simulink model "niof_model"  (R2021a)
settings: Solver=ode23tb  StartTime=0.0  StopTime=2  RelTol=1e-3
values from neighbouring files (symbols this model uses):
  h0 = ds.DateTime(1).Hour + ds.DateTime(1).Minute/60    [compiler_niof_model.m]
  S_area_hole = 0.01    [set_params_blocks.m]
undefined symbols (not defined in the file or in its folder): crop_GH1_NFT_slot1___C, crop_GH1_NFT_slot1___N, crop_GH1_NFT_slot1___R, crop_GH1_NFT_slot2___C, crop_GH1_NFT_slot2___N, crop_GH1_NFT_slot2___R, crop_GH1_NFT_slot3___C, crop_GH1_NFT_slot3___N, crop_GH1_NFT_slot3___R, crop_GH1_NFT_slot4___C, crop_GH1_NFT_slot4___N, crop_GH1_NFT_slot4___R, crop_GH1_RF_slot1___C, crop_GH1_RF_slot1___N, crop_GH1_RF_slot1___R, crop_GH1_RF_slot2___C, crop_GH1_RF_slot2___N, crop_GH1_RF_slot2___R, crop_GH1_RF_slot3___C, crop_GH1_RF_slot3___N, crop_GH1_RF_slot3___R, crop_GH1_RF_slot4___C, crop_GH1_RF_slot4___N, crop_GH1_RF_slot4___R, crop_GH2_RF_slot1___C, crop_GH2_RF_slot1___N, crop_GH2_RF_slot1___R, crop_GH2_RF_slot2___C, crop_GH2_RF_slot2___N, crop_GH2_RF_slot2___R, crop_GH2_RF_slot3___C, crop_GH2_RF_slot3___N, crop_GH2_RF_slot3___R, crop_GH2_RF_slot4___C, crop_GH2_RF_slot4___N, crop_GH2_RF_slot4___R, crop_GH2_TRAD_slot1___C, crop_GH2_TRAD_slot1___N, crop_GH2_TRAD_slot1___R, crop_GH2_TRAD_slot2___C, crop_GH2_TRAD_slot2___N, crop_GH2_TRAD_slot2___R, crop_GH2_TRAD_slot3___C, crop_GH2_TRAD_slot3___N, crop_GH2_TRAD_slot3___R, crop_GH2_TRAD_slot4___C, crop_GH2_TRAD_slot4___N, crop_GH2_TRAD_slot4___R, fish, GH3_Tank1_tend, GH3_Tank2_tend, GH3_Tank3_tend, GH3_Tank4_tend, tp_biofilter___T, tp_fish_C___T, tp_fish_M___T, tp_fish_S___T, tp_fish_T___T, tp_GH1_bio___T, tp_GH1_NFT___T ... (+3)
libraries: HORTISIM x152
(part 2 of 4)

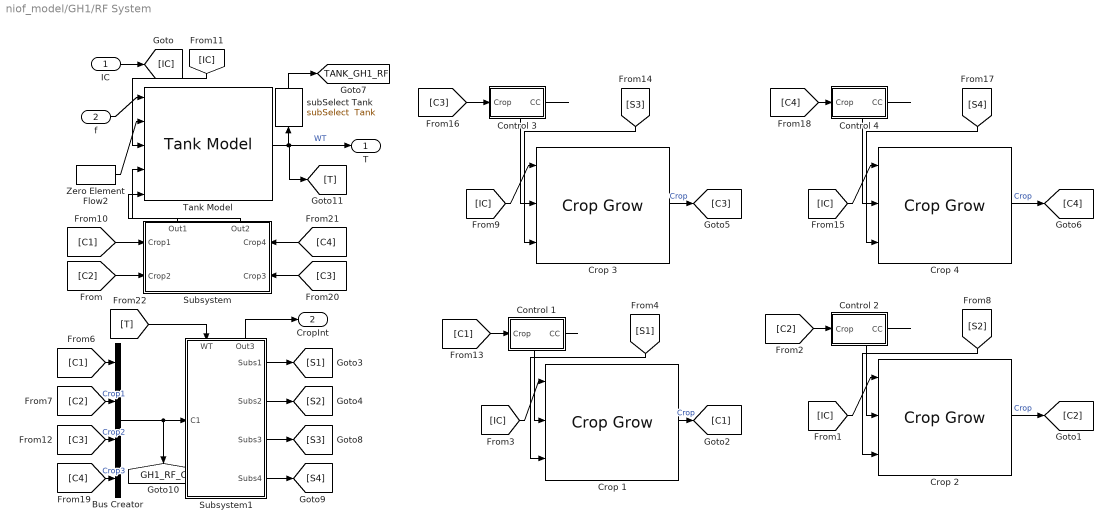
== system niof_model/GH1/RF System ==
  IC : Inport
  f : Inport  Port=2
  Bus Creator : BusCreator  Inputs=4
  Control 1 : Subsystem
  Control 2 : Subsystem
  Control 3 : Subsystem
  Control 4 : Subsystem
  Crop 1 : HORTISIM/Horticulture/Models/Crop Grow  Chi_nutrients=crop_GH1_RF_slot1___Chi_nutrients  A_v=crop_GH1_RF_slot1___A_v  plants_density=crop_GH1_RF_slot1___plants_density  fraction_DM=crop_GH1_RF_slot1___fraction_DM  min_water_capacity=crop_GH1_RF_slot1___min_water_capacity  C_buf_max=crop_GH1_RF_slot1___C_buf_max  T_v_start_fruit=crop_GH1_RF_slot1___T_v_start_fruit  int_air_speed=crop_GH1_RF_slot1___int_air_speed  b_N_uptake=crop_GH1_RF_slot1___b_N_uptake  Tv=crop_GH1_RF_slot1___Tv  C=crop_GH1_RF_slot1___C  R=crop_GH1_RF_slot1___R  Tsum=crop_GH1_RF_slot1___Tsum  C_wv=crop_GH1_RF_slot1___C_wv  N=crop_GH1_RF_slot1___N  rg_fruit=crop_GH1_RF_slot1___rg_fruit  c_fruit_m=crop_GH1_RF_slot1___c_fruit_m  c_fruit_g=crop_GH1_RF_slot1___c_fruit_g  rg_leaf=crop_GH1_RF_slot1___rg_leaf  c_leaf_m=crop_GH1_RF_slot1___c_leaf_m  c_leaf_g=crop_GH1_RF_slot1___c_leaf_g  rg_stem=crop_GH1_RF_slot1___rg_stem  c_stem_m=crop_GH1_RF_slot1___c_stem_m  c_stem_g=crop_GH1_RF_slot1___c_stem_g  VelocityAbsortion=crop_GH1_RF_slot1___VelocityAbsortion  T_max_v=crop_GH1_RF_slot1___T_max_v  s_max_T=crop_GH1_RF_slot1___s_max_T  s_min_T=crop_GH1_RF_slot1___s_min_T  s_buforg_buf=crop_GH1_RF_slot1___s_buforg_buf  T_sum_end=crop_GH1_RF_slot1___T_sum_end  T_max_v24=crop_GH1_RF_slot1___T_max_v24  T_min_v24=crop_GH1_RF_slot1___T_min_v24  s_min_T24=crop_GH1_RF_slot1___s_min_T24  s_max_T24=crop_GH1_RF_slot1___s_max_T24  T_min_v=crop_GH1_RF_slot1___T_min_v
      settings: SourceProductName=Horti Simulator
  Crop 2 : HORTISIM/Horticulture/Models/Crop Grow  Chi_nutrients=crop_GH1_RF_slot2___Chi_nutrients  A_v=crop_GH1_RF_slot2___A_v  plants_density=crop_GH1_RF_slot2___plants_density  fraction_DM=crop_GH1_RF_slot2___fraction_DM  min_water_capacity=crop_GH1_RF_slot2___min_water_capacity  C_buf_max=crop_GH1_RF_slot2___C_buf_max  T_v_start_fruit=crop_GH1_RF_slot2___T_v_start_fruit  int_air_speed=crop_GH1_RF_slot2___int_air_speed  b_N_uptake=crop_GH1_RF_slot2___b_N_uptake  Tv=crop_GH1_RF_slot2___Tv  C=crop_GH1_RF_slot2___C  R=crop_GH1_RF_slot2___R  Tsum=crop_GH1_RF_slot2___Tsum  C_wv=crop_GH1_RF_slot2___C_wv  N=crop_GH1_RF_slot2___N  rg_fruit=crop_GH1_RF_slot2___rg_fruit  c_fruit_m=crop_GH1_RF_slot2___c_fruit_m  c_fruit_g=crop_GH1_RF_slot2___c_fruit_g  rg_leaf=crop_GH1_RF_slot2___rg_leaf  c_leaf_m=crop_GH1_RF_slot2___c_leaf_m  c_leaf_g=crop_GH1_RF_slot2___c_leaf_g  rg_stem=crop_GH1_RF_slot2___rg_stem  c_stem_m=crop_GH1_RF_slot2___c_stem_m  c_stem_g=crop_GH1_RF_slot2___c_stem_g  VelocityAbsortion=crop_GH1_RF_slot2___VelocityAbsortion  T_max_v=crop_GH1_RF_slot2___T_max_v  s_max_T=crop_GH1_RF_slot2___s_max_T  s_min_T=crop_GH1_RF_slot2___s_min_T  s_buforg_buf=crop_GH1_RF_slot2___s_buforg_buf  T_sum_end=crop_GH1_RF_slot2___T_sum_end  T_max_v24=crop_GH1_RF_slot2___T_max_v24  T_min_v24=crop_GH1_RF_slot2___T_min_v24  s_min_T24=crop_GH1_RF_slot2___s_min_T24  s_max_T24=crop_GH1_RF_slot2___s_max_T24  T_min_v=crop_GH1_RF_slot2___T_min_v
      settings: SourceProductName=Horti Simulator
  Crop 3 : HORTISIM/Horticulture/Models/Crop Grow  Chi_nutrients=crop_GH1_RF_slot3___Chi_nutrients  A_v=crop_GH1_RF_slot3___A_v  plants_density=crop_GH1_RF_slot3___plants_density  fraction_DM=crop_GH1_RF_slot3___fraction_DM  min_water_capacity=crop_GH1_RF_slot3___min_water_capacity  C_buf_max=crop_GH1_RF_slot3___C_buf_max  T_v_start_fruit=crop_GH1_RF_slot3___T_v_start_fruit  int_air_speed=crop_GH1_RF_slot3___int_air_speed  b_N_uptake=crop_GH1_RF_slot3___b_N_uptake  Tv=crop_GH1_RF_slot3___Tv  C=crop_GH1_RF_slot3___C  R=crop_GH1_RF_slot3___R  Tsum=crop_GH1_RF_slot3___Tsum  C_wv=crop_GH1_RF_slot3___C_wv  N=crop_GH1_RF_slot3___N  rg_fruit=crop_GH1_RF_slot3___rg_fruit  c_fruit_m=crop_GH1_RF_slot3___c_fruit_m  c_fruit_g=crop_GH1_RF_slot3___c_fruit_g  rg_leaf=crop_GH1_RF_slot3___rg_leaf  c_leaf_m=crop_GH1_RF_slot3___c_leaf_m  c_leaf_g=crop_GH1_RF_slot3___c_leaf_g  rg_stem=crop_GH1_RF_slot3___rg_stem  c_stem_m=crop_GH1_RF_slot3___c_stem_m  c_stem_g=crop_GH1_RF_slot3___c_stem_g  VelocityAbsortion=crop_GH1_RF_slot3___VelocityAbsortion  T_max_v=crop_GH1_RF_slot3___T_max_v  s_max_T=crop_GH1_RF_slot3___s_max_T  s_min_T=crop_GH1_RF_slot3___s_min_T  s_buforg_buf=crop_GH1_RF_slot3___s_buforg_buf  T_sum_end=crop_GH1_RF_slot3___T_sum_end  T_max_v24=crop_GH1_RF_slot3___T_max_v24  T_min_v24=crop_GH1_RF_slot3___T_min_v24  s_min_T24=crop_GH1_RF_slot3___s_min_T24  s_max_T24=crop_GH1_RF_slot3___s_max_T24  T_min_v=crop_GH1_RF_slot3___T_min_v
      settings: SourceProductName=Horti Simulator
  Crop 4 : HORTISIM/Horticulture/Models/Crop Grow  Chi_nutrients=crop_GH1_RF_slot4___Chi_nutrients  A_v=crop_GH1_RF_slot4___A_v  plants_density=crop_GH1_RF_slot4___plants_density  fraction_DM=crop_GH1_RF_slot4___fraction_DM  min_water_capacity=crop_GH1_RF_slot4___min_water_capacity  C_buf_max=crop_GH1_RF_slot4___C_buf_max  T_v_start_fruit=crop_GH1_RF_slot4___T_v_start_fruit  int_air_speed=crop_GH1_RF_slot4___int_air_speed  b_N_uptake=crop_GH1_RF_slot4___b_N_uptake  Tv=crop_GH1_RF_slot4___Tv  C=crop_GH1_RF_slot4___C  R=crop_GH1_RF_slot4___R  Tsum=crop_GH1_RF_slot4___Tsum  C_wv=crop_GH1_RF_slot4___C_wv  N=crop_GH1_RF_slot4___N  rg_fruit=crop_GH1_RF_slot4___rg_fruit  c_fruit_m=crop_GH1_RF_slot4___c_fruit_m  c_fruit_g=crop_GH1_RF_slot4___c_fruit_g  rg_leaf=crop_GH1_RF_slot4___rg_leaf  c_leaf_m=crop_GH1_RF_slot4___c_leaf_m  c_leaf_g=crop_GH1_RF_slot4___c_leaf_g  rg_stem=crop_GH1_RF_slot4___rg_stem  c_stem_m=crop_GH1_RF_slot4___c_stem_m  c_stem_g=crop_GH1_RF_slot4___c_stem_g  VelocityAbsortion=crop_GH1_RF_slot4___VelocityAbsortion  T_max_v=crop_GH1_RF_slot4___T_max_v  s_max_T=crop_GH1_RF_slot4___s_max_T  s_min_T=crop_GH1_RF_slot4___s_min_T  s_buforg_buf=crop_GH1_RF_slot4___s_buforg_buf  T_sum_end=crop_GH1_RF_slot4___T_sum_end  T_max_v24=crop_GH1_RF_slot4___T_max_v24  T_min_v24=crop_GH1_RF_slot4___T_min_v24  s_min_T24=crop_GH1_RF_slot4___s_min_T24  s_max_T24=crop_GH1_RF_slot4___s_max_T24  T_min_v=crop_GH1_RF_slot4___T_min_v
      settings: SourceProductName=Horti Simulator
  Subsystem : Subsystem
      settings: PortSchema="{\"entries\":[{\"content\":{\"sides\":[{\"content\":{\"connectorIds\":[]},\"type\":\"ConnectorPlacement.EquallySpacedRectSide\",\"uuid\":\"331b7e07-99e0-48a1-afa9-efd959d86c3c\"},{\"content\":{\"connectorIds\":[\"Out1\",\"Out2\"],\"side\":\"RIGHT\"},\"type\":\"ConnectorPlacement.EquallySpacedRectSide\",\"uuid\":\"88f560c2-c33d-415c-abbb-9cce13a50e34\"},{\"content\":{\"connectorIds\":[\"In1\",\"In2\"],\"side\":\"TOP\"},\"type\":\"ConnectorPlacement.EquallySpacedRectSide\",\"uuid\":\"5809bd20-6d1a-4a08-a3be-af6196f2651a\"},{\"content\":{\"connectorIds\":[\"In3\",\"In4\"],\"side\":\"BOTTOM\"},\"type\":\"ConnectorPlacement.EquallySpacedRectSide\",\"uuid\":\"0451beb0-e3d9-4028-a291-a4662efcb901\"}]},\"type\":\"ConnectorPlacement.EquallySpacedConnector\",\"uuid\":\"8352e301-80a0-449c-83b8-038a5d79df4c\"}],\"packageUris\":[\"http://schema.mathworks.com/mf0/Connector/R2020b\"],\"version\":\"1.0\"}"
  Subsystem1 : Subsystem
      settings: PortSchema="{\"entries\":[{\"content\":{\"sides\":[{\"content\":{\"connectorIds\":[\"In1\"]},\"type\":\"ConnectorPlacement.EquallySpacedRectSide\",\"uuid\":\"4fbee580-d560-4e1c-bbb5-c1692f8814f1\"},{\"content\":{\"connectorIds\":[\"Out1\",\"Out2\",\"Out3\",\"Out4\"],\"side\":\"RIGHT\"},\"type\":\"ConnectorPlacement.EquallySpacedRectSide\",\"uuid\":\"81a4a23d-0981-460c-8110-0a6c3dae9561\"},{\"content\":{\"connectorIds\":[\"In2\",\"Out5\"],\"side\":\"TOP\"},\"type\":\"ConnectorPlacement.EquallySpacedRectSide\",\"uuid\":\"d86bf355-ad16-490c-942f-99534b60638b\"},{\"content\":{\"connectorIds\":[],\"side\":\"BOTTOM\"},\"type\":\"ConnectorPlacement.EquallySpacedRectSide\",\"uuid\":\"eaa009ab-e9b5-48b4-8c60-43d182c3bfd7\"}]},\"type\":\"ConnectorPlacement.EquallySpacedConnector\",\"uuid\":\"d99c9aa8-04cd-4090-9f71-30da2befe22b\"}],\"packageUris\":[\"http://schema.mathworks.com/mf0/Connector/R2020b\"],\"version\":\"1.0\"}"
  Tank Model : HORTISIM/Aquaculture/Models/Tank Model  S=tp_GH1_RF___S  h_max=tp_GH1_RF___h_max  wall_gain=tp_GH1_RF___wall_gain  ThermalConductivityWall=tp_GH1_RF___ThermalConductivityWall  Tsubwall=tp_GH1_RF___Tsubwall  h=tp_GH1_RF___h  X=tp_GH1_RF___X  T=tp_GH1_RF___T  Twall=tp_GH1_RF___Twall  d_t=tp_GH1_RF___d_t
      settings: SourceProductName=Horti Simulator
  Zero Element Flow2 : HORTISIM/Other  Functions/Zero Element Flow  SystemSampleTime=-1  VariantActivationTime=update diagram  Latency=0  AutoFrameSizeCalculation=off
      settings: SourceProductName=Horti Simulator
  subSelect Tank : HORTISIM/Other  Functions/subSelect  Tank  SystemSampleTime=-1  VariantActivationTime=update diagram  Latency=0  AutoFrameSizeCalculation=off
      settings: SourceProductName=Horti Simulator
  T : Outport
  CropInt : Outport  Port=2
  tag scope: GH1_RF_C=global, TANK_GH1_RF=global
  wires:
  f/1 -> Tank Model/1
  [IC] -> Tank Model/3
  Tank Model/1 -> [T], T/1, subSelect Tank/1  "WT"
  [IC] -> Crop 1/1
  Control 1/1(CC) -> Crop 1/2
  Crop 1/1 -> [C1]  "Crop"
  Zero Element Flow2/1 -> Tank Model/2
  [C1] -> Control 1/1(Crop)
  IC/1 -> [IC]
  [IC] -> Crop 2/1
  Crop 2/1 -> [C2]  "Crop"
  [C2] -> Control 2/1(Crop)
  Control 2/1(CC) -> Crop 2/2
  [S1] -> Crop 1/3
  [S2] -> Crop 2/3
  [C1] -> Subsystem/2(Crop1)
  [C2] -> Subsystem/1(Crop2)
  Subsystem/1(Out1) -> Tank Model/4
  Subsystem/2(Out2) -> Tank Model/5
  [IC] -> Crop 3/1
  Crop 3/1 -> [C3]  "Crop"
  [S3] -> Crop 3/3
  [C3] -> Control 3/1(Crop)
  Control 3/1(CC) -> Crop 3/2
  [IC] -> Crop 4/1
  Crop 4/1 -> [C4]  "Crop"
  [S4] -> Crop 4/3
  [C4] -> Control 4/1(Crop)
  Control 4/1(CC) -> Crop 4/2
  [C3] -> Subsystem/3(Crop3)
  [C4] -> Subsystem/4(Crop4)
  [T] -> Subsystem1/2(WT)
  Subsystem1/1(Subs1) -> [S1]
  Subsystem1/2(Subs2) -> [S2]
  Subsystem1/5(Out3) -> CropInt/1
  Subsystem1/3(Subs3) -> [S3]
  Subsystem1/4(Subs4) -> [S4]
  [C1] -> Bus Creator/1
  [C2] -> Bus Creator/2  "Crop1"
  [C3] -> Bus Creator/3  "Crop2"
  [C4] -> Bus Creator/4  "Crop3"
  Bus Creator/1 -> [GH1_RF_C], Subsystem1/1(C1)
  subSelect Tank/1 -> [TANK_GH1_RF]

== system niof_model/GH1/Subsystem ==
  In1 : Inport
  In2 : Inport  Port=2
  In3 : Inport  Port=3
  In4 : Inport  Port=4
  Crop2ExtArray : HORTISIM/Other  Functions/Crop2ExtArray  SystemSampleTime=-1  VariantActivationTime=update diagram  Latency=0  AutoFrameSizeCalculation=off
      settings: SourceProductName=Horti Simulator
  Crop2ExtArray1 : HORTISIM/Other  Functions/Crop2ExtArray  SystemSampleTime=-1  VariantActivationTime=update diagram  Latency=0  AutoFrameSizeCalculation=off
      settings: SourceProductName=Horti Simulator
  MatrixExt2Bus : HORTISIM/Other  Functions/MatrixExt2Bus  SystemSampleTime=-1  VariantActivationTime=update diagram  Latency=0  AutoFrameSizeCalculation=off
      settings: SourceProductName=Horti Simulator
  Tank2ExtArray : HORTISIM/Other  Functions/Tank2ExtArray  SystemSampleTime=-1  VariantActivationTime=update diagram  Latency=0  AutoFrameSizeCalculation=off
      settings: SourceProductName=Horti Simulator
  Tank2ExtArray1 : HORTISIM/Other  Functions/Tank2ExtArray  SystemSampleTime=-1  VariantActivationTime=update diagram  Latency=0  AutoFrameSizeCalculation=off
      settings: SourceProductName=Horti Simulator
  Vector Concatenate : Concatenate  NumInputs=4  Mode=Multidimensional array  ConcatenateDimension=2
  CoCl : Outport
  wires:
  MatrixExt2Bus/1 -> CoCl/1
  In2/1 -> Tank2ExtArray/1
  Crop2ExtArray1/1 -> Vector Concatenate/4
  In1/1 -> Crop2ExtArray/1
  In3/1 -> Tank2ExtArray1/1
  Tank2ExtArray1/1 -> Vector Concatenate/3
  In4/1 -> Crop2ExtArray1/1
  Vector Concatenate/1 -> MatrixExt2Bus/1
  Tank2ExtArray/1 -> Vector Concatenate/2
  Crop2ExtArray/1 -> Vector Concatenate/1

== system niof_model/GH1/Subsystem1 ==
  In1 : Inport
  In2 : Inport  Port=2
  Bus Selector : BusSelector  OutputSignals=Drainge
  Bus Selector1 : BusSelector  OutputSignals=Drainge
  Subsystem3 : Subsystem
  Out1 : Outport
  wires:
  In2/1 -> Bus Selector1/1
  In1/1 -> Bus Selector/1
  Bus Selector/1 -> Subsystem3/1(In1)  "<Drainge>"
  Subsystem3/1(Out1) -> Out1/1
  Bus Selector1/1 -> Subsystem3/2(In2)  "<Drainge>"

== system niof_model/GH2/Flow2Divisor ==
  Fo2 : Inport
  In1 : Inport  Port=2
  Bus Creator : BusCreator  Inputs=3  OutDataTypeStr=Bus: FLOW  NonVirtualBus=on
  Bus Creator1 : BusCreator  Inputs=3  OutDataTypeStr=Bus: FLOW  NonVirtualBus=on
  Bus Selector : BusSelector  OutputSignals=f,T,X
  Constant : Constant
  Minus : Sum  Inputs=+-
  Product : Product
  Product1 : Product
  Out1 : Outport
  Out2 : Outport  Port=2
  wires:
  Fo2/1 -> Bus Selector/1
  Bus Selector/1 -> Product1/2, Product/2  "<f>"
  Product/1 -> [f1]
  Bus Selector/2 -> [T]  "<T>"
  Bus Selector/3 -> [X]  "<X>"
  [f1] -> Bus Creator/1  "f"
  [T] -> Bus Creator/2  "T"
  Bus Creator/1 -> Out1/1
  [X] -> Bus Creator/3  "X"
  [f2] -> Bus Creator1/1  "f"
  [T] -> Bus Creator1/2  "T"
  Bus Creator1/1 -> Out2/1
  [X] -> Bus Creator1/3  "X"
  In1/1 -> Product/1, Minus/2
  Constant/1 -> Minus/1
  Minus/1 -> Product1/1
  Product1/1 -> [f2]

== system niof_model/GH2/Mezcla Calor, Vapor de agua y CO2 desde los tanques de agua y la plantación ==
  In2 : Inport
  In3 : Inport  Port=2
  In4 : Inport  Port=3
  In1 : Inport  Port=4
  Crop2ExtArray : Subsystem  AncestorBlock="HORTISIM/Other  Functions/Crop2ExtArray"
  Crop2ExtArray1 : HORTISIM/Other  Functions/Crop2ExtArray  SystemSampleTime=-1  VariantActivationTime=update diagram  Latency=0  AutoFrameSizeCalculation=off
      settings: SourceProductName=Horti Simulator
  MatrixExt2Bus : Subsystem  AncestorBlock="HORTISIM/Other  Functions/MatrixExt2Bus"
  Tank2ExtArray : Subsystem  AncestorBlock="HORTISIM/Other  Functions/Tank2ExtArray"
  Tank2ExtArray1 : HORTISIM/Other  Functions/Tank2ExtArray  SystemSampleTime=-1  VariantActivationTime=update diagram  Latency=0  AutoFrameSizeCalculation=off
      settings: SourceProductName=Horti Simulator
  Vector Concatenate : Concatenate  NumInputs=4  Mode=Multidimensional array  ConcatenateDimension=2
  CoCl : Outport
  wires:
  In4/1 -> Crop2ExtArray1/1
  In3/1 -> Tank2ExtArray1/1
  In2/1 -> Tank2ExtArray/1(In1)
  Crop2ExtArray/1(Out1) -> Vector Concatenate/1
  Vector Concatenate/1 -> MatrixExt2Bus/1(In1)
  MatrixExt2Bus/1(CoCl) -> CoCl/1
  Tank2ExtArray/1(Out1) -> Vector Concatenate/2
  Tank2ExtArray1/1 -> Vector Concatenate/3
  Crop2ExtArray1/1 -> Vector Concatenate/4
  In1/1 -> Crop2ExtArray/1(In1)

== system niof_model/GH2/Null Element ==
  Scalar2Bus Control Climate : HORTISIM/Other  Functions/Scalar2Bus  Control Climate  SystemSampleTime=-1  VariantActivationTime=update diagram  Latency=0  AutoFrameSizeCalculation=off
      settings: SourceProductName=Horti Simulator
  Zero Element Screen : HORTISIM/Other  Functions/Zero Element Screen  SystemSampleTime=-1  VariantActivationTime=update diagram  Latency=0  AutoFrameSizeCalculation=off
      settings: SourceProductName=Horti Simulator
  Zero Element Windows : HORTISIM/Other  Functions/Zero Element Windows  SystemSampleTime=-1  VariantActivationTime=update diagram  Latency=0  AutoFrameSizeCalculation=off
      link override Constant1: Value=1
      settings: SourceProductName=Horti Simulator
  CoCl : Outport
  wires:
  Scalar2Bus Control Climate/1 -> CoCl/1
  Zero Element Windows/1 -> Scalar2Bus Control Climate/1
  ? -> Scalar2Bus Control Climate/4
  ? -> Scalar2Bus Control Climate/3
  Zero Element Screen/1 -> Scalar2Bus Control Climate/2

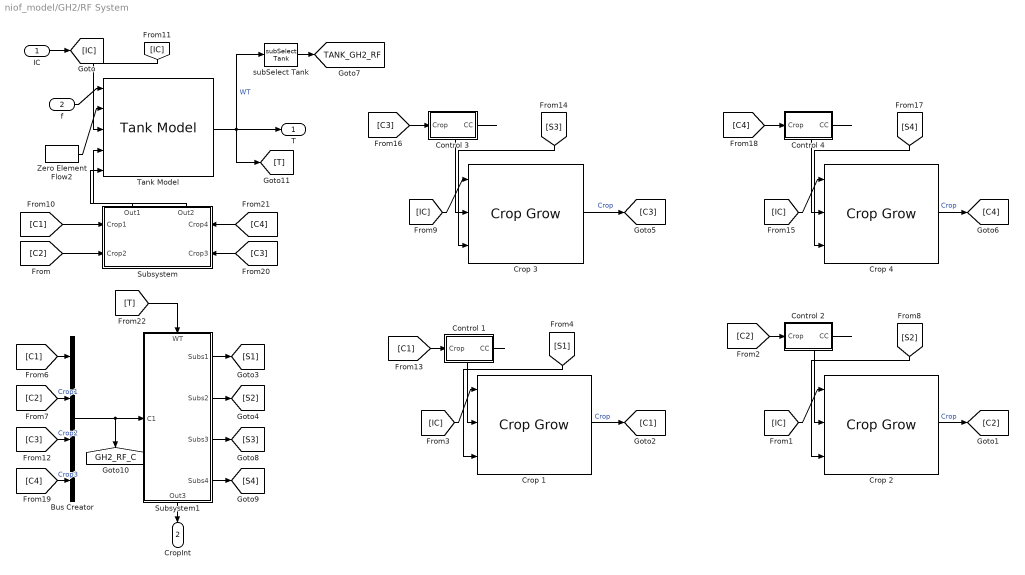
== system niof_model/GH2/RF System ==
  IC : Inport
  f : Inport  Port=2
  Bus Creator : BusCreator  Inputs=4
  Control 1 : Subsystem
  Control 2 : Subsystem
  Control 3 : Subsystem
  Control 4 : Subsystem
  Crop 1 : HORTISIM/Horticulture/Models/Crop Grow  Chi_nutrients=crop_GH2_RF_slot1___Chi_nutrients  A_v=crop_GH2_RF_slot1___A_v  plants_density=crop_GH2_RF_slot1___plants_density  fraction_DM=crop_GH2_RF_slot1___fraction_DM  min_water_capacity=crop_GH2_RF_slot1___min_water_capacity  C_buf_max=crop_GH2_RF_slot1___C_buf_max  T_v_start_fruit=crop_GH2_RF_slot1___T_v_start_fruit  int_air_speed=crop_GH2_RF_slot1___int_air_speed  b_N_uptake=crop_GH2_RF_slot1___b_N_uptake  Tv=crop_GH2_RF_slot1___Tv  C=crop_GH2_RF_slot1___C  R=crop_GH2_RF_slot1___R  Tsum=crop_GH2_RF_slot1___Tsum  C_wv=crop_GH2_RF_slot1___C_wv  N=crop_GH2_RF_slot1___N  rg_fruit=crop_GH2_RF_slot1___rg_fruit  c_fruit_m=crop_GH2_RF_slot1___c_fruit_m  c_fruit_g=crop_GH2_RF_slot1___c_fruit_g  rg_leaf=crop_GH2_RF_slot1___rg_leaf  c_leaf_m=crop_GH2_RF_slot1___c_leaf_m  c_leaf_g=crop_GH2_RF_slot1___c_leaf_g  rg_stem=crop_GH2_RF_slot1___rg_stem  c_stem_m=crop_GH2_RF_slot1___c_stem_m  c_stem_g=crop_GH2_RF_slot1___c_stem_g  VelocityAbsortion=crop_GH2_RF_slot1___VelocityAbsortion  T_max_v=crop_GH2_RF_slot1___T_max_v  s_max_T=crop_GH2_RF_slot1___s_max_T  s_min_T=crop_GH2_RF_slot1___s_min_T  s_buforg_buf=crop_GH2_RF_slot1___s_buforg_buf  T_sum_end=crop_GH2_RF_slot1___T_sum_end  T_max_v24=crop_GH2_RF_slot1___T_max_v24  T_min_v24=crop_GH2_RF_slot1___T_min_v24  s_min_T24=crop_GH2_RF_slot1___s_min_T24  s_max_T24=crop_GH2_RF_slot1___s_max_T24  T_min_v=crop_GH2_RF_slot1___T_min_v
      settings: SourceProductName=Horti Simulator
  Crop 2 : HORTISIM/Horticulture/Models/Crop Grow  Chi_nutrients=crop_GH2_RF_slot2___Chi_nutrients  A_v=crop_GH2_RF_slot2___A_v  plants_density=crop_GH2_RF_slot2___plants_density  fraction_DM=crop_GH2_RF_slot2___fraction_DM  min_water_capacity=crop_GH2_RF_slot2___min_water_capacity  C_buf_max=crop_GH2_RF_slot2___C_buf_max  T_v_start_fruit=crop_GH2_RF_slot2___T_v_start_fruit  int_air_speed=crop_GH2_RF_slot2___int_air_speed  b_N_uptake=crop_GH2_RF_slot2___b_N_uptake  Tv=crop_GH2_RF_slot2___Tv  C=crop_GH2_RF_slot2___C  R=crop_GH2_RF_slot2___R  Tsum=crop_GH2_RF_slot2___Tsum  C_wv=crop_GH2_RF_slot2___C_wv  N=crop_GH2_RF_slot2___N  rg_fruit=crop_GH2_RF_slot2___rg_fruit  c_fruit_m=crop_GH2_RF_slot2___c_fruit_m  c_fruit_g=crop_GH2_RF_slot2___c_fruit_g  rg_leaf=crop_GH2_RF_slot2___rg_leaf  c_leaf_m=crop_GH2_RF_slot2___c_leaf_m  c_leaf_g=crop_GH2_RF_slot2___c_leaf_g  rg_stem=crop_GH2_RF_slot2___rg_stem  c_stem_m=crop_GH2_RF_slot2___c_stem_m  c_stem_g=crop_GH2_RF_slot2___c_stem_g  VelocityAbsortion=crop_GH2_RF_slot2___VelocityAbsortion  T_max_v=crop_GH2_RF_slot2___T_max_v  s_max_T=crop_GH2_RF_slot2___s_max_T  s_min_T=crop_GH2_RF_slot2___s_min_T  s_buforg_buf=crop_GH2_RF_slot2___s_buforg_buf  T_sum_end=crop_GH2_RF_slot2___T_sum_end  T_max_v24=crop_GH2_RF_slot2___T_max_v24  T_min_v24=crop_GH2_RF_slot2___T_min_v24  s_min_T24=crop_GH2_RF_slot2___s_min_T24  s_max_T24=crop_GH2_RF_slot2___s_max_T24  T_min_v=crop_GH2_RF_slot2___T_min_v
      settings: SourceProductName=Horti Simulator
  Crop 3 : HORTISIM/Horticulture/Models/Crop Grow  Chi_nutrients=crop_GH2_RF_slot3___Chi_nutrients  A_v=crop_GH2_RF_slot3___A_v  plants_density=crop_GH2_RF_slot3___plants_density  fraction_DM=crop_GH2_RF_slot3___fraction_DM  min_water_capacity=crop_GH2_RF_slot3___min_water_capacity  C_buf_max=crop_GH2_RF_slot3___C_buf_max  T_v_start_fruit=crop_GH2_RF_slot3___T_v_start_fruit  int_air_speed=crop_GH2_RF_slot3___int_air_speed  b_N_uptake=crop_GH2_RF_slot3___b_N_uptake  Tv=crop_GH2_RF_slot3___Tv  C=crop_GH2_RF_slot3___C  R=crop_GH2_RF_slot3___R  Tsum=crop_GH2_RF_slot3___Tsum  C_wv=crop_GH2_RF_slot3___C_wv  N=crop_GH2_RF_slot3___N  rg_fruit=crop_GH2_RF_slot3___rg_fruit  c_fruit_m=crop_GH2_RF_slot3___c_fruit_m  c_fruit_g=crop_GH2_RF_slot3___c_fruit_g  rg_leaf=crop_GH2_RF_slot3___rg_leaf  c_leaf_m=crop_GH2_RF_slot3___c_leaf_m  c_leaf_g=crop_GH2_RF_slot3___c_leaf_g  rg_stem=crop_GH2_RF_slot3___rg_stem  c_stem_m=crop_GH2_RF_slot3___c_stem_m  c_stem_g=crop_GH2_RF_slot3___c_stem_g  VelocityAbsortion=crop_GH2_RF_slot3___VelocityAbsortion  T_max_v=crop_GH2_RF_slot3___T_max_v  s_max_T=crop_GH2_RF_slot3___s_max_T  s_min_T=crop_GH2_RF_slot3___s_min_T  s_buforg_buf=crop_GH2_RF_slot3___s_buforg_buf  T_sum_end=crop_GH2_RF_slot3___T_sum_end  T_max_v24=crop_GH2_RF_slot3___T_max_v24  T_min_v24=crop_GH2_RF_slot3___T_min_v24  s_min_T24=crop_GH2_RF_slot3___s_min_T24  s_max_T24=crop_GH2_RF_slot3___s_max_T24  T_min_v=crop_GH2_RF_slot3___T_min_v
      settings: SourceProductName=Horti Simulator
  Crop 4 : HORTISIM/Horticulture/Models/Crop Grow  Chi_nutrients=crop_GH2_RF_slot4___Chi_nutrients  A_v=crop_GH2_RF_slot4___A_v  plants_density=crop_GH2_RF_slot4___plants_density  fraction_DM=crop_GH2_RF_slot4___fraction_DM  min_water_capacity=crop_GH2_RF_slot4___min_water_capacity  C_buf_max=crop_GH2_RF_slot4___C_buf_max  T_v_start_fruit=crop_GH2_RF_slot4___T_v_start_fruit  int_air_speed=crop_GH2_RF_slot4___int_air_speed  b_N_uptake=crop_GH2_RF_slot4___b_N_uptake  Tv=crop_GH2_RF_slot4___Tv  C=crop_GH2_RF_slot4___C  R=crop_GH2_RF_slot4___R  Tsum=crop_GH2_RF_slot4___Tsum  C_wv=crop_GH2_RF_slot4___C_wv  N=crop_GH2_RF_slot4___N  rg_fruit=crop_GH2_RF_slot4___rg_fruit  c_fruit_m=crop_GH2_RF_slot4___c_fruit_m  c_fruit_g=crop_GH2_RF_slot4___c_fruit_g  rg_leaf=crop_GH2_RF_slot4___rg_leaf  c_leaf_m=crop_GH2_RF_slot4___c_leaf_m  c_leaf_g=crop_GH2_RF_slot4___c_leaf_g  rg_stem=crop_GH2_RF_slot4___rg_stem  c_stem_m=crop_GH2_RF_slot4___c_stem_m  c_stem_g=crop_GH2_RF_slot4___c_stem_g  VelocityAbsortion=crop_GH2_RF_slot4___VelocityAbsortion  T_max_v=crop_GH2_RF_slot4___T_max_v  s_max_T=crop_GH2_RF_slot4___s_max_T  s_min_T=crop_GH2_RF_slot4___s_min_T  s_buforg_buf=crop_GH2_RF_slot4___s_buforg_buf  T_sum_end=crop_GH2_RF_slot4___T_sum_end  T_max_v24=crop_GH2_RF_slot4___T_max_v24  T_min_v24=crop_GH2_RF_slot4___T_min_v24  s_min_T24=crop_GH2_RF_slot4___s_min_T24  s_max_T24=crop_GH2_RF_slot4___s_max_T24  T_min_v=crop_GH2_RF_slot4___T_min_v
      settings: SourceProductName=Horti Simulator
  Subsystem : Subsystem
      settings: PortSchema="{\"entries\":[{\"content\":{\"sides\":[{\"content\":{\"connectorIds\":[]},\"type\":\"ConnectorPlacement.EquallySpacedRectSide\",\"uuid\":\"331b7e07-99e0-48a1-afa9-efd959d86c3c\"},{\"content\":{\"connectorIds\":[\"Out1\",\"Out2\"],\"side\":\"RIGHT\"},\"type\":\"ConnectorPlacement.EquallySpacedRectSide\",\"uuid\":\"88f560c2-c33d-415c-abbb-9cce13a50e34\"},{\"content\":{\"connectorIds\":[\"In1\",\"In2\"],\"side\":\"TOP\"},\"type\":\"ConnectorPlacement.EquallySpacedRectSide\",\"uuid\":\"5809bd20-6d1a-4a08-a3be-af6196f2651a\"},{\"content\":{\"connectorIds\":[\"In3\",\"In4\"],\"side\":\"BOTTOM\"},\"type\":\"ConnectorPlacement.EquallySpacedRectSide\",\"uuid\":\"0451beb0-e3d9-4028-a291-a4662efcb901\"}]},\"type\":\"ConnectorPlacement.EquallySpacedConnector\",\"uuid\":\"8352e301-80a0-449c-83b8-038a5d79df4c\"}],\"packageUris\":[\"http://schema.mathworks.com/mf0/Connector/R2020b\"],\"version\":\"1.0\"}"
  Subsystem1 : Subsystem
      settings: PortSchema="{\"entries\":[{\"content\":{\"sides\":[{\"content\":{\"connectorIds\":[\"In1\"]},\"type\":\"ConnectorPlacement.EquallySpacedRectSide\",\"uuid\":\"4fbee580-d560-4e1c-bbb5-c1692f8814f1\"},{\"content\":{\"connectorIds\":[\"Out1\",\"Out2\",\"Out3\",\"Out4\"],\"side\":\"RIGHT\"},\"type\":\"ConnectorPlacement.EquallySpacedRectSide\",\"uuid\":\"81a4a23d-0981-460c-8110-0a6c3dae9561\"},{\"content\":{\"connectorIds\":[\"In2\"],\"side\":\"TOP\"},\"type\":\"ConnectorPlacement.EquallySpacedRectSide\",\"uuid\":\"d86bf355-ad16-490c-942f-99534b60638b\"},{\"content\":{\"connectorIds\":[\"Out5\"],\"side\":\"BOTTOM\"},\"type\":\"ConnectorPlacement.EquallySpacedRectSide\",\"uuid\":\"eaa009ab-e9b5-48b4-8c60-43d182c3bfd7\"}]},\"type\":\"ConnectorPlacement.EquallySpacedConnector\",\"uuid\":\"d99c9aa8-04cd-4090-9f71-30da2befe22b\"}],\"packageUris\":[\"http://schema.mathworks.com/mf0/Connector/R2020b\"],\"version\":\"1.0\"}"
  Tank Model : HORTISIM/Aquaculture/Models/Tank Model  S=tp_GH2_RF___S  h_max=tp_GH2_RF___h_max  wall_gain=tp_GH2_RF___wall_gain  ThermalConductivityWall=tp_GH2_RF___ThermalConductivityWall  Tsubwall=tp_GH2_RF___Tsubwall  h=tp_GH2_RF___h  X=tp_GH2_RF___X  T=tp_GH2_RF___T  Twall=tp_GH2_RF___Twall  d_t=tp_GH2_RF___d_t
      settings: SourceProductName=Horti Simulator
  Zero Element Flow2 : HORTISIM/Other  Functions/Zero Element Flow  SystemSampleTime=-1  VariantActivationTime=update diagram  Latency=0  AutoFrameSizeCalculation=off
      settings: SourceProductName=Horti Simulator
  subSelect Tank : HORTISIM/Other  Functions/subSelect  Tank  SystemSampleTime=-1  VariantActivationTime=update diagram  Latency=0  AutoFrameSizeCalculation=off
      settings: SourceProductName=Horti Simulator
  T : Outport
  CropInt : Outport  Port=2
  tag scope: GH2_RF_C=global, TANK_GH2_RF=global
  wires:
  f/1 -> Tank Model/1
  [IC] -> Tank Model/3
  Tank Model/1 -> T/1, [T], subSelect Tank/1  "WT"
  [IC] -> Crop 1/1
  Control 1/1(CC) -> Crop 1/2
  Crop 1/1 -> [C1]  "Crop"
  Zero Element Flow2/1 -> Tank Model/2
  [C1] -> Control 1/1(Crop)
  IC/1 -> [IC]
  [IC] -> Crop 2/1
  Crop 2/1 -> [C2]  "Crop"
  [C2] -> Control 2/1(Crop)
  Control 2/1(CC) -> Crop 2/2
  [S1] -> Crop 1/3
  [S2] -> Crop 2/3
  [C1] -> Subsystem/2(Crop1)
  [C2] -> Subsystem/1(Crop2)
  Subsystem/1(Out1) -> Tank Model/4
  Subsystem/2(Out2) -> Tank Model/5
  [IC] -> Crop 3/1
  Crop 3/1 -> [C3]  "Crop"
  [S3] -> Crop 3/3
  [C3] -> Control 3/1(Crop)
  Control 3/1(CC) -> Crop 3/2
  [IC] -> Crop 4/1
  Crop 4/1 -> [C4]  "Crop"
  [S4] -> Crop 4/3
  [C4] -> Control 4/1(Crop)
  Control 4/1(CC) -> Crop 4/2
  [C3] -> Subsystem/3(Crop3)
  [C4] -> Subsystem/4(Crop4)
  [T] -> Subsystem1/2(WT)
  Subsystem1/1(Subs1) -> [S1]
  Subsystem1/2(Subs2) -> [S2]
  Subsystem1/5(Out3) -> CropInt/1
  Subsystem1/3(Subs3) -> [S3]
  Subsystem1/4(Subs4) -> [S4]
  [C1] -> Bus Creator/1
  [C2] -> Bus Creator/2  "Crop1"
  [C3] -> Bus Creator/3  "Crop2"
  [C4] -> Bus Creator/4  "Crop3"
  Bus Creator/1 -> [GH2_RF_C], Subsystem1/1(C1)
  subSelect Tank/1 -> [TANK_GH2_RF]

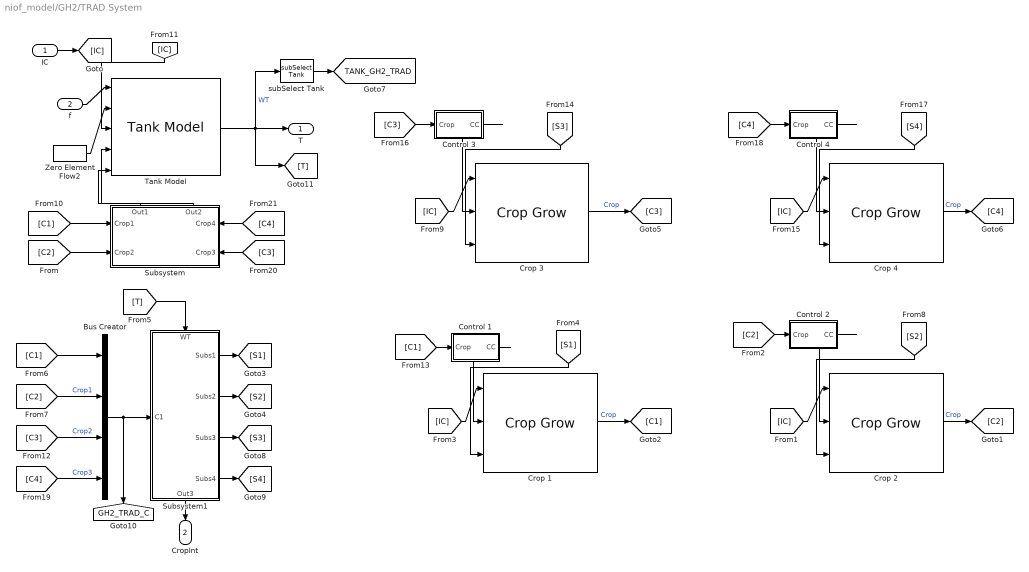
== system niof_model/GH2/TRAD System ==
  IC : Inport
  f : Inport  Port=2
  Bus Creator : BusCreator  Inputs=4
  Control 1 : Subsystem
  Control 2 : Subsystem
  Control 3 : Subsystem
  Control 4 : Subsystem
  Crop 1 : HORTISIM/Horticulture/Models/Crop Grow  Chi_nutrients=crop_GH2_TRAD_slot1___Chi_nutrients  A_v=crop_GH2_TRAD_slot1___A_v  plants_density=crop_GH2_TRAD_slot1___plants_density  fraction_DM=crop_GH2_TRAD_slot1___fraction_DM  min_water_capacity=crop_GH2_TRAD_slot1___min_water_capacity  C_buf_max=crop_GH2_TRAD_slot1___C_buf_max  T_v_start_fruit=crop_GH2_TRAD_slot1___T_v_start_fruit  int_air_speed=crop_GH2_TRAD_slot1___int_air_speed  b_N_uptake=crop_GH2_TRAD_slot1___b_N_uptake  Tv=crop_GH2_TRAD_slot1___Tv  C=crop_GH2_TRAD_slot1___C  R=crop_GH2_TRAD_slot1___R  Tsum=crop_GH2_TRAD_slot1___Tsum  C_wv=crop_GH2_TRAD_slot1___C_wv  N=crop_GH2_TRAD_slot1___N  rg_fruit=crop_GH2_TRAD_slot1___rg_fruit  c_fruit_m=crop_GH2_TRAD_slot1___c_fruit_m  c_fruit_g=crop_GH2_TRAD_slot1___c_fruit_g  rg_leaf=crop_GH2_TRAD_slot1___rg_leaf  c_leaf_m=crop_GH2_TRAD_slot1___c_leaf_m  c_leaf_g=crop_GH2_TRAD_slot1___c_leaf_g  rg_stem=crop_GH2_TRAD_slot1___rg_stem  c_stem_m=crop_GH2_TRAD_slot1___c_stem_m  c_stem_g=crop_GH2_TRAD_slot1___c_stem_g  VelocityAbsortion=crop_GH2_TRAD_slot1___VelocityAbsortion  T_max_v=crop_GH2_TRAD_slot1___T_max_v  s_max_T=crop_GH2_TRAD_slot1___s_max_T  s_min_T=crop_GH2_TRAD_slot1___s_min_T  s_buforg_buf=crop_GH2_TRAD_slot1___s_buforg_buf  T_sum_end=crop_GH2_TRAD_slot1___T_sum_end  T_max_v24=crop_GH2_TRAD_slot1___T_max_v24  T_min_v24=crop_GH2_TRAD_slot1___T_min_v24  s_min_T24=crop_GH2_TRAD_slot1___s_min_T24  s_max_T24=crop_GH2_TRAD_slot1___s_max_T24  T_min_v=crop_GH2_TRAD_slot1___T_min_v
      settings: SourceProductName=Horti Simulator
  Crop 2 : HORTISIM/Horticulture/Models/Crop Grow  Chi_nutrients=crop_GH2_TRAD_slot2___Chi_nutrients  A_v=crop_GH2_TRAD_slot2___A_v  plants_density=crop_GH2_TRAD_slot2___plants_density  fraction_DM=crop_GH2_TRAD_slot2___fraction_DM  min_water_capacity=crop_GH2_TRAD_slot2___min_water_capacity  C_buf_max=crop_GH2_TRAD_slot2___C_buf_max  T_v_start_fruit=crop_GH2_TRAD_slot2___T_v_start_fruit  int_air_speed=crop_GH2_TRAD_slot2___int_air_speed  b_N_uptake=crop_GH2_TRAD_slot2___b_N_uptake  Tv=crop_GH2_TRAD_slot2___Tv  C=crop_GH2_TRAD_slot2___C  R=crop_GH2_TRAD_slot2___R  Tsum=crop_GH2_TRAD_slot2___Tsum  C_wv=crop_GH2_TRAD_slot2___C_wv  N=crop_GH2_TRAD_slot2___N  rg_fruit=crop_GH2_TRAD_slot2___rg_fruit  c_fruit_m=crop_GH2_TRAD_slot2___c_fruit_m  c_fruit_g=crop_GH2_TRAD_slot2___c_fruit_g  rg_leaf=crop_GH2_TRAD_slot2___rg_leaf  c_leaf_m=crop_GH2_TRAD_slot2___c_leaf_m  c_leaf_g=crop_GH2_TRAD_slot2___c_leaf_g  rg_stem=crop_GH2_TRAD_slot2___rg_stem  c_stem_m=crop_GH2_TRAD_slot2___c_stem_m  c_stem_g=crop_GH2_TRAD_slot2___c_stem_g  VelocityAbsortion=crop_GH2_TRAD_slot2___VelocityAbsortion  T_max_v=crop_GH2_TRAD_slot2___T_max_v  s_max_T=crop_GH2_TRAD_slot2___s_max_T  s_min_T=crop_GH2_TRAD_slot2___s_min_T  s_buforg_buf=crop_GH2_TRAD_slot2___s_buforg_buf  T_sum_end=crop_GH2_TRAD_slot2___T_sum_end  T_max_v24=crop_GH2_TRAD_slot2___T_max_v24  T_min_v24=crop_GH2_TRAD_slot2___T_min_v24  s_min_T24=crop_GH2_TRAD_slot2___s_min_T24  s_max_T24=crop_GH2_TRAD_slot2___s_max_T24  T_min_v=crop_GH2_TRAD_slot2___T_min_v
      settings: SourceProductName=Horti Simulator
  Crop 3 : HORTISIM/Horticulture/Models/Crop Grow  Chi_nutrients=crop_GH2_TRAD_slot3___Chi_nutrients  A_v=crop_GH2_TRAD_slot3___A_v  plants_density=crop_GH2_TRAD_slot3___plants_density  fraction_DM=crop_GH2_TRAD_slot3___fraction_DM  min_water_capacity=crop_GH2_TRAD_slot3___min_water_capacity  C_buf_max=crop_GH2_TRAD_slot3___C_buf_max  T_v_start_fruit=crop_GH2_TRAD_slot3___T_v_start_fruit  int_air_speed=crop_GH2_TRAD_slot3___int_air_speed  b_N_uptake=crop_GH2_TRAD_slot3___b_N_uptake  Tv=crop_GH2_TRAD_slot3___Tv  C=crop_GH2_TRAD_slot3___C  R=crop_GH2_TRAD_slot3___R  Tsum=crop_GH2_TRAD_slot3___Tsum  C_wv=crop_GH2_TRAD_slot3___C_wv  N=crop_GH2_TRAD_slot3___N  rg_fruit=crop_GH2_TRAD_slot3___rg_fruit  c_fruit_m=crop_GH2_TRAD_slot3___c_fruit_m  c_fruit_g=crop_GH2_TRAD_slot3___c_fruit_g  rg_leaf=crop_GH2_TRAD_slot3___rg_leaf  c_leaf_m=crop_GH2_TRAD_slot3___c_leaf_m  c_leaf_g=crop_GH2_TRAD_slot3___c_leaf_g  rg_stem=crop_GH2_TRAD_slot3___rg_stem  c_stem_m=crop_GH2_TRAD_slot3___c_stem_m  c_stem_g=crop_GH2_TRAD_slot3___c_stem_g  VelocityAbsortion=crop_GH2_TRAD_slot3___VelocityAbsortion  T_max_v=crop_GH2_TRAD_slot3___T_max_v  s_max_T=crop_GH2_TRAD_slot3___s_max_T  s_min_T=crop_GH2_TRAD_slot3___s_min_T  s_buforg_buf=crop_GH2_TRAD_slot3___s_buforg_buf  T_sum_end=crop_GH2_TRAD_slot3___T_sum_end  T_max_v24=crop_GH2_TRAD_slot3___T_max_v24  T_min_v24=crop_GH2_TRAD_slot3___T_min_v24  s_min_T24=crop_GH2_TRAD_slot3___s_min_T24  s_max_T24=crop_GH2_TRAD_slot3___s_max_T24  T_min_v=crop_GH2_TRAD_slot3___T_min_v
      settings: SourceProductName=Horti Simulator
  Crop 4 : HORTISIM/Horticulture/Models/Crop Grow  Chi_nutrients=crop_GH2_TRAD_slot4___Chi_nutrients  A_v=crop_GH2_TRAD_slot4___A_v  plants_density=crop_GH2_TRAD_slot4___plants_density  fraction_DM=crop_GH2_TRAD_slot4___fraction_DM  min_water_capacity=crop_GH2_TRAD_slot4___min_water_capacity  C_buf_max=crop_GH2_TRAD_slot4___C_buf_max  T_v_start_fruit=crop_GH2_TRAD_slot4___T_v_start_fruit  int_air_speed=crop_GH2_TRAD_slot4___int_air_speed  b_N_uptake=crop_GH2_TRAD_slot4___b_N_uptake  Tv=crop_GH2_TRAD_slot4___Tv  C=crop_GH2_TRAD_slot4___C  R=crop_GH2_TRAD_slot4___R  Tsum=crop_GH2_TRAD_slot4___Tsum  C_wv=crop_GH2_TRAD_slot4___C_wv  N=crop_GH2_TRAD_slot4___N  rg_fruit=crop_GH2_TRAD_slot4___rg_fruit  c_fruit_m=crop_GH2_TRAD_slot4___c_fruit_m  c_fruit_g=crop_GH2_TRAD_slot4___c_fruit_g  rg_leaf=crop_GH2_TRAD_slot4___rg_leaf  c_leaf_m=crop_GH2_TRAD_slot4___c_leaf_m  c_leaf_g=crop_GH2_TRAD_slot4___c_leaf_g  rg_stem=crop_GH2_TRAD_slot4___rg_stem  c_stem_m=crop_GH2_TRAD_slot4___c_stem_m  c_stem_g=crop_GH2_TRAD_slot4___c_stem_g  VelocityAbsortion=crop_GH2_TRAD_slot4___VelocityAbsortion  T_max_v=crop_GH2_TRAD_slot4___T_max_v  s_max_T=crop_GH2_TRAD_slot4___s_max_T  s_min_T=crop_GH2_TRAD_slot4___s_min_T  s_buforg_buf=crop_GH2_TRAD_slot4___s_buforg_buf  T_sum_end=crop_GH2_TRAD_slot4___T_sum_end  T_max_v24=crop_GH2_TRAD_slot4___T_max_v24  T_min_v24=crop_GH2_TRAD_slot4___T_min_v24  s_min_T24=crop_GH2_TRAD_slot4___s_min_T24  s_max_T24=crop_GH2_TRAD_slot4___s_max_T24  T_min_v=crop_GH2_TRAD_slot4___T_min_v
      settings: SourceProductName=Horti Simulator
  Subsystem : Subsystem
      settings: PortSchema="{\"entries\":[{\"content\":{\"sides\":[{\"content\":{\"connectorIds\":[]},\"type\":\"ConnectorPlacement.EquallySpacedRectSide\",\"uuid\":\"331b7e07-99e0-48a1-afa9-efd959d86c3c\"},{\"content\":{\"connectorIds\":[\"Out1\",\"Out2\"],\"side\":\"RIGHT\"},\"type\":\"ConnectorPlacement.EquallySpacedRectSide\",\"uuid\":\"88f560c2-c33d-415c-abbb-9cce13a50e34\"},{\"content\":{\"connectorIds\":[\"In1\",\"In2\"],\"side\":\"TOP\"},\"type\":\"ConnectorPlacement.EquallySpacedRectSide\",\"uuid\":\"5809bd20-6d1a-4a08-a3be-af6196f2651a\"},{\"content\":{\"connectorIds\":[\"In3\",\"In4\"],\"side\":\"BOTTOM\"},\"type\":\"ConnectorPlacement.EquallySpacedRectSide\",\"uuid\":\"0451beb0-e3d9-4028-a291-a4662efcb901\"}]},\"type\":\"ConnectorPlacement.EquallySpacedConnector\",\"uuid\":\"8352e301-80a0-449c-83b8-038a5d79df4c\"}],\"packageUris\":[\"http://schema.mathworks.com/mf0/Connector/R2020b\"],\"version\":\"1.0\"}"
  Subsystem1 : Subsystem
      settings: PortSchema="{\"entries\":[{\"content\":{\"sides\":[{\"content\":{\"connectorIds\":[\"In1\"]},\"type\":\"ConnectorPlacement.EquallySpacedRectSide\",\"uuid\":\"4fbee580-d560-4e1c-bbb5-c1692f8814f1\"},{\"content\":{\"connectorIds\":[\"Out1\",\"Out2\",\"Out3\",\"Out4\"],\"side\":\"RIGHT\"},\"type\":\"ConnectorPlacement.EquallySpacedRectSide\",\"uuid\":\"81a4a23d-0981-460c-8110-0a6c3dae9561\"},{\"content\":{\"connectorIds\":[\"In2\"],\"side\":\"TOP\"},\"type\":\"ConnectorPlacement.EquallySpacedRectSide\",\"uuid\":\"d86bf355-ad16-490c-942f-99534b60638b\"},{\"content\":{\"connectorIds\":[\"Out5\"],\"side\":\"BOTTOM\"},\"type\":\"ConnectorPlacement.EquallySpacedRectSide\",\"uuid\":\"eaa009ab-e9b5-48b4-8c60-43d182c3bfd7\"}]},\"type\":\"ConnectorPlacement.EquallySpacedConnector\",\"uuid\":\"d99c9aa8-04cd-4090-9f71-30da2befe22b\"}],\"packageUris\":[\"http://schema.mathworks.com/mf0/Connector/R2020b\"],\"version\":\"1.0\"}"
  Tank Model : HORTISIM/Aquaculture/Models/Tank Model  S=tp_GH2_TRAD___S  h_max=tp_GH2_TRAD___h_max  wall_gain=tp_GH2_TRAD___wall_gain  ThermalConductivityWall=tp_GH2_TRAD___ThermalConductivityWall  Tsubwall=tp_GH2_TRAD___Tsubwall  h=tp_GH2_TRAD___h  X=tp_GH2_TRAD___X  T=tp_GH2_TRAD___T  Twall=tp_GH2_TRAD___Twall  d_t=tp_GH2_TRAD___d_t
      settings: SourceProductName=Horti Simulator
  Zero Element Flow2 : HORTISIM/Other  Functions/Zero Element Flow  SystemSampleTime=-1  VariantActivationTime=update diagram  Latency=0  AutoFrameSizeCalculation=off
      settings: SourceProductName=Horti Simulator
  subSelect Tank : HORTISIM/Other  Functions/subSelect  Tank  SystemSampleTime=-1  VariantActivationTime=update diagram  Latency=0  AutoFrameSizeCalculation=off
      settings: SourceProductName=Horti Simulator
  T : Outport
  CropInt : Outport  Port=2
  tag scope: GH2_TRAD_C=global, TANK_GH2_TRAD=global
  wires:
  f/1 -> Tank Model/1
  [IC] -> Tank Model/3
  Tank Model/1 -> subSelect Tank/1, [T], T/1  "WT"
  [IC] -> Crop 1/1
  Control 1/1(CC) -> Crop 1/2
  Crop 1/1 -> [C1]  "Crop"
  Zero Element Flow2/1 -> Tank Model/2
  [C1] -> Control 1/1(Crop)
  IC/1 -> [IC]
  [IC] -> Crop 2/1
  Crop 2/1 -> [C2]  "Crop"
  [C2] -> Control 2/1(Crop)
  Control 2/1(CC) -> Crop 2/2
  [S1] -> Crop 1/3
  [S2] -> Crop 2/3
  [C1] -> Subsystem/2(Crop1)
  [C2] -> Subsystem/1(Crop2)
  Subsystem/1(Out1) -> Tank Model/4
  Subsystem/2(Out2) -> Tank Model/5
  [IC] -> Crop 3/1
  Crop 3/1 -> [C3]  "Crop"
  [S3] -> Crop 3/3
  [C3] -> Control 3/1(Crop)
  Control 3/1(CC) -> Crop 3/2
  [IC] -> Crop 4/1
  Crop 4/1 -> [C4]  "Crop"
  [S4] -> Crop 4/3
  [C4] -> Control 4/1(Crop)
  Control 4/1(CC) -> Crop 4/2
  [C3] -> Subsystem/3(Crop3)
  [C4] -> Subsystem/4(Crop4)
  [T] -> Subsystem1/2(WT)
  Subsystem1/1(Subs1) -> [S1]
  Subsystem1/2(Subs2) -> [S2]
  Subsystem1/5(Out3) -> CropInt/1
  Subsystem1/3(Subs3) -> [S3]
  Subsystem1/4(Subs4) -> [S4]
  [C1] -> Bus Creator/1
  [C2] -> Bus Creator/2  "Crop1"
  [C3] -> Bus Creator/3  "Crop2"
  [C4] -> Bus Creator/4  "Crop3"
  Bus Creator/1 -> Subsystem1/1(C1), [GH2_TRAD_C]
  subSelect Tank/1 -> [TANK_GH2_TRAD]

== system niof_model/GH2/add drainge flows ==
  In1 : Inport
  In2 : Inport  Port=2
  Abs : Abs  ZeroCross=off
  Bus Creator : BusCreator  Inputs=3  OutDataTypeStr=Bus: FLOW  NonVirtualBus=on
  Bus Selector : BusSelector  OutputSignals=Drainge
  Bus Selector1 : BusSelector  OutputSignals=Drainge
  Bus Selector2 : BusSelector  OutputSignals=f
  Bus Selector3 : BusSelector  OutputSignals=f
  If : If  IfExpression=u1 <1e-8
  If Action Subsystem : Subsystem  TreatAsAtomicUnit=on
  If Action Subsystem1 : Subsystem  TreatAsAtomicUnit=on
  Merge : Merge
  Merge1 : Merge
  Merge2 : Merge
  Sum : Sum  Inputs=|++
  Out1 : Outport
  wires:
  In2/1 -> Bus Selector1/1
  In1/1 -> Bus Selector/1
  Bus Creator/1 -> Out1/1
  Bus Selector/1 -> [F1], Bus Selector2/1  "<Drainge>"
  Bus Selector1/1 -> [F2], Bus Selector3/1  "<Drainge>"
  If/2 -> If Action Subsystem1/Action
  Merge2/1 -> Bus Creator/3  "X"
  Merge1/1 -> Bus Creator/2  "T"
  Merge/1 -> Bus Creator/1  "f"
  If Action Subsystem/1(f) -> Merge/1
  If Action Subsystem1/1(f) -> Merge/2
  If Action Subsystem/2(T) -> Merge1/1
  If Action Subsystem1/2(T) -> Merge1/2
  If Action Subsystem/3(X) -> Merge2/1
  If Action Subsystem1/3(X) -> Merge2/2
  [F1] -> If Action Subsystem1/1(In1)
  [F2] -> If Action Subsystem1/2(In2)
  [F1] -> If Action Subsystem/1(In1)
  If/1 -> If Action Subsystem/Action
  Abs/1 -> If/1
  Sum/1 -> Abs/1
  [f2] -> Sum/2
  [f1] -> Sum/1
  Bus Selector3/1 -> [f2]  "<f>"
  Bus Selector2/1 -> [f1]  "<f>"

== system niof_model/GH3/Air Pump ==
  note: %N K Ca Mg P S O2 TSS
  Constant : Constant  Value=[0 0 0 0 0 0 1 0]'  VectorParams1D=off
  Gain : Gain
  Out Bus Element : Outport  PortName=O2  Element=R
  wires:
  Constant/1 -> Gain/1
  Gain/1 -> Out Bus Element/1

== system niof_model/GH3/Comunication Vessels ==
  In Bus Element : Inport  PortName=WT1  Element=h
  In Bus Element2 : Inport  PortName=WT1  Element=Fout.T
  In Bus Element4 : Inport  PortName=WT1  Element=Fout.X
  In Bus Element1 : Inport  Port=2  PortName=WT2  Element=h
  In Bus Element3 : Inport  Port=2  PortName=WT2  Element=Fout.T
  In Bus Element5 : Inport  Port=2  PortName=WT2  Element=Fout.X
  Bus Creator : BusCreator  Inputs=3  OutDataTypeStr=Bus: FLOW  NonVirtualBus=on
  Bus Creator1 : BusCreator  Inputs=3  OutDataTypeStr=Bus: FLOW  NonVirtualBus=on
  Gain : Gain  Gain=2*9.8*S
  Gain1 : Gain  Gain=-1
  Minus : Sum  Inputs=+-
  F12 : Outport
  F21 : Outport  Port=2
  wires:
  In Bus Element/1 -> Minus/1
  In Bus Element1/1 -> Minus/2
  Minus/1 -> Gain/1
  Gain/1 -> [FLOW]
  Bus Creator/1 -> F12/1
  [FLOW] -> Bus Creator/1  "f"
  In Bus Element2/1 -> Bus Creator/2  "T"
  In Bus Element4/1 -> Bus Creator/3  "X"
  Bus Creator1/1 -> F21/1
  Gain1/1 -> Bus Creator1/1  "f"
  In Bus Element3/1 -> Bus Creator1/2  "T"
  In Bus Element5/1 -> Bus Creator1/3  "X"
  [FLOW] -> Gain1/1  "f"

== system niof_model/GH3/Comunication Vessels1 ==
  In Bus Element : Inport  PortName=WT1  Element=h
  In Bus Element2 : Inport  PortName=WT1  Element=Fout.T
  In Bus Element4 : Inport  PortName=WT1  Element=Fout.X
  In Bus Element1 : Inport  Port=2  PortName=WT2  Element=h
  In Bus Element3 : Inport  Port=2  PortName=WT2  Element=Fout.T
  In Bus Element5 : Inport  Port=2  PortName=WT2  Element=Fout.X
  Bus Creator : BusCreator  Inputs=3  OutDataTypeStr=Bus: FLOW  NonVirtualBus=on
  Bus Creator1 : BusCreator  Inputs=3  OutDataTypeStr=Bus: FLOW  NonVirtualBus=on
  Gain : Gain  Gain=2*9.8*S
  Gain1 : Gain  Gain=-1
  Minus : Sum  Inputs=+-
  F12 : Outport
  F21 : Outport  Port=2
  wires:
  In Bus Element/1 -> Minus/1
  In Bus Element1/1 -> Minus/2
  Minus/1 -> Gain/1
  Gain/1 -> [FLOW]
  Bus Creator/1 -> F12/1
  [FLOW] -> Bus Creator/1  "f"
  In Bus Element2/1 -> Bus Creator/2  "T"
  In Bus Element4/1 -> Bus Creator/3  "X"
  Bus Creator1/1 -> F21/1
  Gain1/1 -> Bus Creator1/1  "f"
  In Bus Element3/1 -> Bus Creator1/2  "T"
  In Bus Element5/1 -> Bus Creator1/3  "X"
  [FLOW] -> Gain1/1  "f"

== system niof_model/GH3/Comunication Vessels2 ==
  In Bus Element : Inport  PortName=WT1  Element=h
  In Bus Element2 : Inport  PortName=WT1  Element=Fout.T
  In Bus Element4 : Inport  PortName=WT1  Element=Fout.X
  In Bus Element1 : Inport  Port=2  PortName=WT2  Element=h
  In Bus Element3 : Inport  Port=2  PortName=WT2  Element=Fout.T
  In Bus Element5 : Inport  Port=2  PortName=WT2  Element=Fout.X
  Bus Creator : BusCreator  Inputs=3  OutDataTypeStr=Bus: FLOW  NonVirtualBus=on
  Bus Creator1 : BusCreator  Inputs=3  OutDataTypeStr=Bus: FLOW  NonVirtualBus=on
  Gain : Gain  Gain=2*9.8*S
  Gain1 : Gain  Gain=-1
  Minus : Sum  Inputs=+-
  F12 : Outport
  F21 : Outport  Port=2
  wires:
  In Bus Element/1 -> Minus/1
  In Bus Element1/1 -> Minus/2
  Minus/1 -> Gain/1
  Gain/1 -> [FLOW]
  Bus Creator/1 -> F12/1
  [FLOW] -> Bus Creator/1  "f"
  In Bus Element2/1 -> Bus Creator/2  "T"
  In Bus Element4/1 -> Bus Creator/3  "X"
  Bus Creator1/1 -> F21/1
  Gain1/1 -> Bus Creator1/1  "f"
  In Bus Element3/1 -> Bus Creator1/2  "T"
  In Bus Element5/1 -> Bus Creator1/3  "X"
  [FLOW] -> Gain1/1  "f"

== system niof_model/GH3/Null Element ==
  Scalar2Bus Control Climate : HORTISIM/Other  Functions/Scalar2Bus  Control Climate  SystemSampleTime=-1  VariantActivationTime=update diagram  Latency=0  AutoFrameSizeCalculation=off
      settings: SourceProductName=Horti Simulator
  Zero Element Screen : HORTISIM/Other  Functions/Zero Element Screen  SystemSampleTime=-1  VariantActivationTime=update diagram  Latency=0  AutoFrameSizeCalculation=off
      settings: SourceProductName=Horti Simulator
  Zero Element Windows : HORTISIM/Other  Functions/Zero Element Windows  SystemSampleTime=-1  VariantActivationTime=update diagram  Latency=0  AutoFrameSizeCalculation=off
      link override Constant1: Value=1
      settings: SourceProductName=Horti Simulator
  CoCl : Outport
  wires:
  Scalar2Bus Control Climate/1 -> CoCl/1
  Zero Element Windows/1 -> Scalar2Bus Control Climate/1
  ? -> Scalar2Bus Control Climate/4
  ? -> Scalar2Bus Control Climate/3
  Zero Element Screen/1 -> Scalar2Bus Control Climate/2

== system niof_model/GH3/Subsystem ==
  In3 : Inport
  In4 : Inport  Port=2
  In2 : Inport  Port=3
  In1 : Inport  Port=4
  Bus Selector{1..4} (4 alike) : BusSelector  OutputSignals=QV,QT
  "Scalar2Bus Ext Signal " : HORTISIM/Other  Functions/Scalar2Bus Ext Signal    SystemSampleTime=-1  VariantActivationTime=update diagram  Latency=0  AutoFrameSizeCalculation=off
      settings: SourceProductName=Horti Simulator
  Sum : Sum  Inputs=++++
  Sum1 : Sum  Inputs=++++
  CoCl : Outport
  wires:
  ? -> "Scalar2Bus Ext Signal "/3
  ? -> "Scalar2Bus Ext Signal "/4
  In2/1 -> Bus Selector1/1
  "Scalar2Bus Ext Signal "/1 -> CoCl/1
  In3/1 -> Bus Selector2/1
  In1/1 -> Bus Selector3/1
  In4/1 -> Bus Selector4/1
  Sum/1 -> "Scalar2Bus Ext Signal "/1
  Bus Selector3/1 -> Sum/1  "<QV>"
  Bus Selector1/1 -> Sum/2  "<QV>"
  Bus Selector2/1 -> Sum/3  "<QV>"
  Bus Selector4/1 -> Sum/4  "<QV>"
  Bus Selector3/2 -> Sum1/1  "<QT>"
  Bus Selector1/2 -> Sum1/2  "<QT>"
  Bus Selector2/2 -> Sum1/3  "<QT>"
  Bus Selector4/2 -> Sum1/4  "<QT>"
  Sum1/1 -> "Scalar2Bus Ext Signal "/2

== system niof_model/GH3/Subsystem1 ==
  FT : Inport
  O2 : Inport  Port=2
  Bus Selector1 : BusSelector  OutputSignals=R
  Bus Selector2 : BusSelector  OutputSignals=R
  Vector Concatenate2 : Concatenate  Mode=Multidimensional array  ConcatenateDimension=2
  R : Outport
  wires:
  FT/1 -> Bus Selector1/1
  Bus Selector2/1 -> Vector Concatenate2/2  "<R>"
  O2/1 -> Bus Selector2/1
  Vector Concatenate2/1 -> R/1
  Bus Selector1/1 -> Vector Concatenate2/1  "<R>"

== system niof_model/GH3/Subsystem2 ==
  FT : Inport
  O2 : Inport  Port=2
  Bus Selector1 : BusSelector  OutputSignals=R
  Bus Selector2 : BusSelector  OutputSignals=R
  Vector Concatenate2 : Concatenate  Mode=Multidimensional array  ConcatenateDimension=2
  R : Outport
  wires:
  FT/1 -> Bus Selector1/1
  Bus Selector2/1 -> Vector Concatenate2/2  "<R>"
  O2/1 -> Bus Selector2/1
  Vector Concatenate2/1 -> R/1
  Bus Selector1/1 -> Vector Concatenate2/1  "<R>"

== system niof_model/GH3/Subsystem3 ==
  note: Well Water1
  Bus Creator1 : BusCreator  Inputs=3  OutDataTypeStr=Bus: FLOW  NonVirtualBus=on
  "[Kelvin]1" : Constant  Value=273.15 + 20
  kg/m^1 : Constant  Value=1 + zeros(8,1)
  "m^3{H2O}/s1" : Constant  Value=0
  Fin : Outport
  wires:
  Bus Creator1/1 -> Fin/1
  kg/m^1/1 -> Bus Creator1/3  "X"
  "[Kelvin]1"/1 -> Bus Creator1/2  "T"
  "m^3{H2O}/s1"/1 -> Bus Creator1/1  "f"

== system niof_model/GH3/Subsystem4 ==
  note: Well Water1
  Bus Creator1 : BusCreator  Inputs=3  OutDataTypeStr=Bus: FLOW  NonVirtualBus=on
  "[Kelvin]1" : Constant  Value=273.15 + 20
  kg/m^1 : Constant  Value=1 + zeros(8,1)
  "m^3{H2O}/s1" : Constant  Value=0
  Fin : Outport
  wires:
  Bus Creator1/1 -> Fin/1
  kg/m^1/1 -> Bus Creator1/3  "X"
  "[Kelvin]1"/1 -> Bus Creator1/2  "T"
  "m^3{H2O}/s1"/1 -> Bus Creator1/1  "f"

== system niof_model/GH3/Subsystem5 ==
  FT : Inport
  O2 : Inport  Port=2
  Bus Selector1 : BusSelector  OutputSignals=R
  Bus Selector2 : BusSelector  OutputSignals=R
  Vector Concatenate2 : Concatenate  Mode=Multidimensional array  ConcatenateDimension=2
  R : Outport
  wires:
  FT/1 -> Bus Selector1/1
  Bus Selector2/1 -> Vector Concatenate2/2  "<R>"
  O2/1 -> Bus Selector2/1
  Vector Concatenate2/1 -> R/1
  Bus Selector1/1 -> Vector Concatenate2/1  "<R>"

== system niof_model/GH3/Subsystem6 ==
  Mass : Inport
  Bus Selector : BusSelector  OutputSignals=dmdt
  Feed Convertio Ratio : Gain  Gain=FCR
  Product : Product
  Pulse Generator : DiscretePulseGenerator  PulseType=Time based  Period=1  PulseWidth=5
  Feed : Outport
  wires:
  Mass/1 -> Bus Selector/1
  Bus Selector/1 -> Feed Convertio Ratio/1  "<dmdt>"
  Feed Convertio Ratio/1 -> Product/2
  Product/1 -> Feed/1
  Pulse Generator/1 -> Product/1

== system niof_model/GH3/Subsystem7 ==
  FT : Inport
  O2 : Inport  Port=2
  Bus Selector1 : BusSelector  OutputSignals=R
  Bus Selector2 : BusSelector  OutputSignals=R
  Vector Concatenate2 : Concatenate  Mode=Multidimensional array  ConcatenateDimension=2
  R : Outport
  wires:
  FT/1 -> Bus Selector1/1
  Bus Selector2/1 -> Vector Concatenate2/2  "<R>"
  O2/1 -> Bus Selector2/1
  Vector Concatenate2/1 -> R/1
  Bus Selector1/1 -> Vector Concatenate2/1  "<R>"

== system niof_model/GH3/Tank1 ==
  Start/Stop Window : HORTISIM/Other  Functions/Start//Stop Window  tinit=GH3_Tank1_tinit  tend=GH3_Tank1_tend
      settings: SourceProductName=Horti Simulator
  Out1 : Outport
  wires:
  Start/Stop Window/1 -> Out1/1

== system niof_model/GH3/Tank2 ==
  Start/Stop Window : HORTISIM/Other  Functions/Start//Stop Window  tinit=GH3_Tank2_tinit  tend=GH3_Tank2_tend
      settings: SourceProductName=Horti Simulator
  Out1 : Outport
  wires:
  Start/Stop Window/1 -> Out1/1

== system niof_model/GH3/Tank3 ==
  Start/Stop Window : HORTISIM/Other  Functions/Start//Stop Window  tinit=GH3_Tank3_tinit  tend=GH3_Tank3_tend
      settings: SourceProductName=Horti Simulator
  Out1 : Outport
  wires:
  Start/Stop Window/1 -> Out1/1

== system niof_model/GH3/Tank4 ==
  Start/Stop Window : HORTISIM/Other  Functions/Start//Stop Window  tinit=GH3_Tank4_tinit  tend=GH3_Tank4_tend
      settings: SourceProductName=Horti Simulator
  Out1 : Outport
  wires:
  Start/Stop Window/1 -> Out1/1

== system niof_model/GH3/Zero Element Flow ==
  note: Well Water1
  Bus Creator1 : BusCreator  Inputs=3  OutDataTypeStr=Bus: FLOW  NonVirtualBus=on
  "[Kelvin]1" : Constant  Value=273.15 + 20
  kg/m^1 : Constant  Value=1 + zeros(8,1)
  "m^3{H2O}/s1" : Constant  Value=0
  Fin : Outport
  wires:
  Bus Creator1/1 -> Fin/1
  kg/m^1/1 -> Bus Creator1/3  "X"
  "[Kelvin]1"/1 -> Bus Creator1/2  "T"
  "m^3{H2O}/s1"/1 -> Bus Creator1/1  "f"
